simulink model "Copy_of_Feedbak_linearization"  (R2023a)
settings: Solver=VariableStepAuto  StartTime=0.0  StopTime=150  RelTol=1e-3
InitFcn:
  | FL_init
values from neighbouring files (symbols this model uses):
  dz0 = 0    [FL_init.m]
  g = 9.81    [FL_init.m]    (also in INIT_R.m)
  I = 1/3*m*L^2    (= 0.666666666667)    [INIT_R.m]
  L = 1    [INIT_R.m]
  m = 0.261    [FL_init.m]    (also in INIT_R.m = 2)
settings Model: Creator=rvitt  LastModifiedBy=rvitt

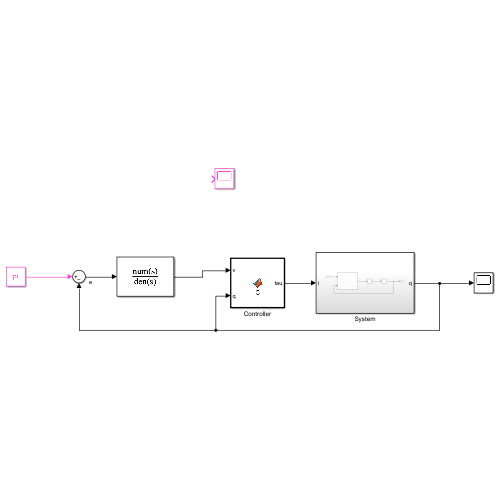
[thumbnail: Simulink's stored preview of the top-level diagram]
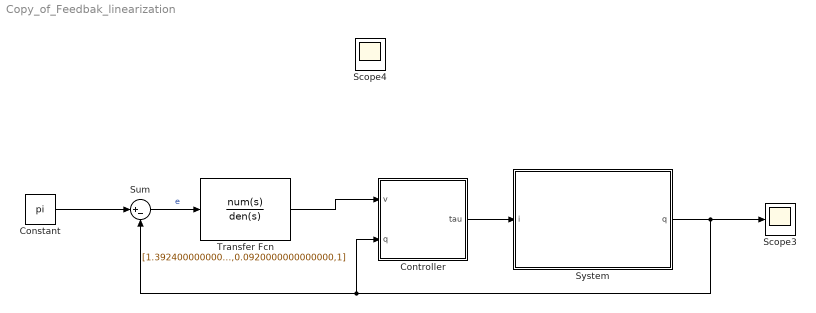
== system Copy_of_Feedbak_linearization ==
  Constant : Constant  Value=pi
  Controller : MATLAB Function  TreatAsAtomicUnit=on
  Scope3 : Scope
  Scope4 : Scope
  Sum : Sum  Inputs=|+-
  System : Subsystem
  Transfer Fcn : TransferFcn  Numerator=[1.39240000000000,2.36000000000000,1]  Denominator=[0.00211600000000000,0.0920000000000000,1]
  wires:
  System/1(q) -> Scope3/1, Controller/2(q), Sum/2
  Constant/1 -> Sum/1
  Controller/1(tau) -> System/1(i)
  Transfer Fcn/1 -> Controller/1(v)
  Sum/1 -> Transfer Fcn/1  "e"

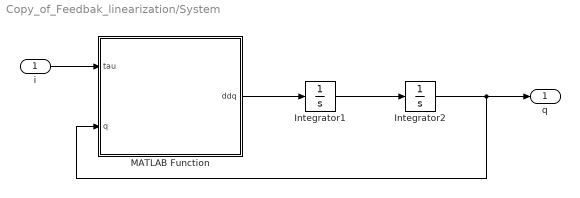
== system Copy_of_Feedbak_linearization/System ==
  i : Inport
  Integrator1 : Integrator  InitialCondition=dz0
  Integrator2 : Integrator
  MATLAB Function : MATLAB Function  TreatAsAtomicUnit=on
  q : Outport
  wires:
  i/1 -> MATLAB Function/1(tau)
  Integrator1/1 -> Integrator2/1
  Integrator2/1 -> q/1, MATLAB Function/2(q)
  MATLAB Function/1(ddq) -> Integrator1/1

== matlab function Copy_of_Feedbak_linearization/Controller ==
  data: m parameter; v input; g parameter; q input; tau output; I parameter; L parameter
function tau = C(m, v, g, q, I, L)

tau = m*g*L*sin(q) + I*v;

== matlab function Copy_of_Feedbak_linearization/System/MATLAB Function ==
  data: tau input; m parameter; g parameter; q input; ddq output; L parameter; I parameter
function ddq  = model(tau, m, g, q, L, I)

% System dynamics 
ddq = (tau - m*g*sin(q)*L)/I;
